simulink model "vienna_car_part2"  (R2019b)
settings: Solver=VariableStepAuto  StartTime=0.0  StopTime=100  RelTol=1e-3
values from neighbouring files (symbols this model uses):
  simulation_length_track = distance_A_B    [main.m]
  slope_of_track = 3    [main.m]
undefined symbols (not defined in the file or in its folder): air_density, drag_coefficient, equ_mass_of_rot_parts, gravity, mass, rolling_resistance_coefficient_0, rolling_resistance_coefficient_1, surface_area, wheel_radius
settings Model: Creator=jamil  LastModifiedBy=jamil
settings SolverCC: ZeroCrossAlgorithm=Adaptive
settings DebuggingCC: IgnoredZcDiagnostic=none

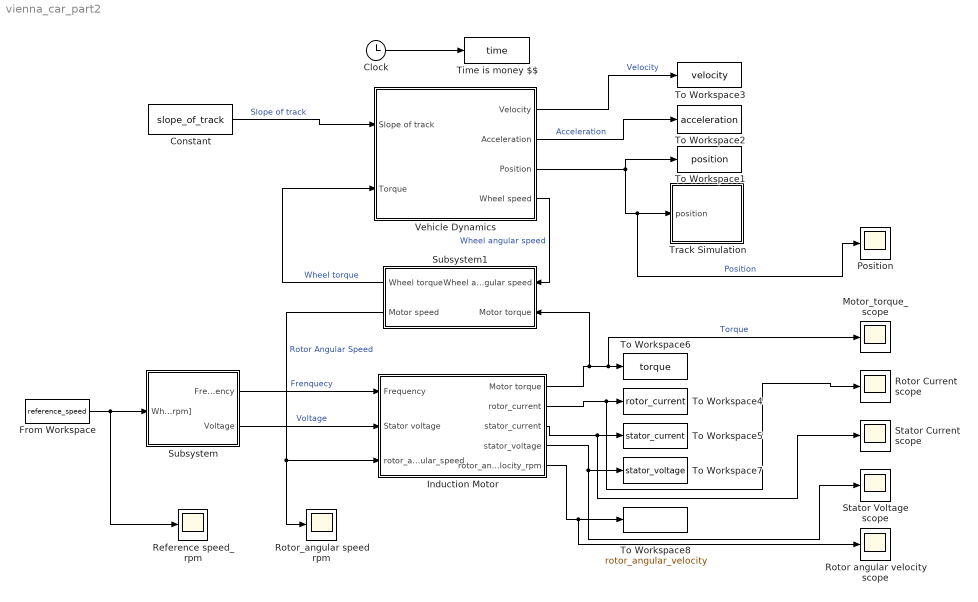
== system vienna_car_part2 ==
  Clock : Clock
  Constant : Constant  Value=slope_of_track
  From Workspace : FromWorkspace  VariableName=reference_speed  SampleTime=0
  Induction Motor : Subsystem
      mask Display: image('induction_motor_pic.jpg')
  Motor_torque_scope : Scope
  Position : Scope
  Reference speed_rpm : Scope
  "Rotor Current scope " : Scope
  Rotor angular velocity scope : Scope
  Rotor_angular speed rpm : Scope
  Stator Current scope : Scope
  Stator Voltage scope : Scope
  Subsystem : Subsystem
      mask Display: image('variable_speed_drive_pic.png')
  Subsystem1 : Subsystem
      mask Display: image('gearbox_pic.jpg'); % Use "Edit Image" on toolstrip to change.
  Time is money $$ : ToWorkspace  VariableName=time  SampleTime=-1
  To Workspace1 : ToWorkspace  VariableName=position  SampleTime=-1
  To Workspace2 : ToWorkspace  VariableName=acceleration  SampleTime=-1
  To Workspace3 : ToWorkspace  VariableName=velocity  SampleTime=-1
  To Workspace4 : ToWorkspace  VariableName=rotor_current  SampleTime=-1
  To Workspace5 : ToWorkspace  VariableName=stator_current  SampleTime=-1
  To Workspace6 : ToWorkspace  VariableName=torque  SampleTime=-1
  To Workspace7 : ToWorkspace  VariableName=stator_voltage  SampleTime=-1
  To Workspace8 : ToWorkspace  VariableName=rotor_angular_velocity  SampleTime=-1
  Track Simulation : Subsystem
  Vehicle Dynamics : Subsystem
      mask Display: image('car_dynamic_pic.jpg'); % Use "Edit Image" on toolstrip to change.
  wires:
  Vehicle Dynamics/2(Acceleration) -> To Workspace2/1  "Acceleration"
  Vehicle Dynamics/3(Position) -> Position/1, Track Simulation/1(position), To Workspace1/1  "Position"
  Constant/1 -> Vehicle Dynamics/1("Slope of track ")  "Slope of track"
  Vehicle Dynamics/1(Velocity) -> To Workspace3/1  "Velocity"
  Clock/1 -> Time is money $$/1
  Subsystem1/2(Motor speed) -> Rotor_angular speed rpm/1, Induction Motor/3("rotor_angular_speed ")  "Rotor Angular Speed"
  Induction Motor/1(Motor torque) -> Subsystem1/2(Motor torque), Motor_torque_scope/1, To Workspace6/1  "Torque"
  Subsystem/1(Frequency) -> Induction Motor/1("Frequency ")  "Frenquecy"
  Subsystem/2(Voltage) -> Induction Motor/2("Stator voltage ")  "Voltage"
  From Workspace/1 -> Reference speed_rpm/1, Subsystem/1(Wheel speed [rpm])
  Induction Motor/4(stator_voltage) -> Stator Voltage scope/1, To Workspace7/1
  Induction Motor/5(rotor_angular_velocity_rpm) -> Rotor angular velocity scope/1, To Workspace8/1
  Induction Motor/2(rotor_current) -> "Rotor Current scope "/1, To Workspace4/1
  Induction Motor/3(stator_current) -> Stator Current scope/1, To Workspace5/1
  Vehicle Dynamics/4(Wheel speed) -> Subsystem1/1(Wheel angular speed)  "Wheel angular speed"
  Subsystem1/1("Wheel torque ") -> Vehicle Dynamics/2(Torque)  "Wheel torque"

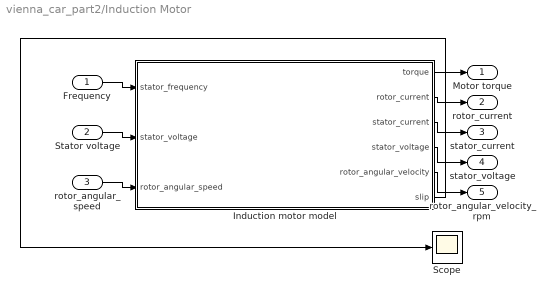
== system vienna_car_part2/Induction Motor ==
  "Frequency " : Inport
  "Stator voltage " : Inport  Port=2
  "rotor_angular_speed " : Inport  Port=3
  "Induction motor model " : MATLAB Function  TreatAsAtomicUnit=on
  Scope : Scope
  Motor torque : Outport
  rotor_current : Outport  Port=2
  stator_current : Outport  Port=3
  stator_voltage : Outport  Port=4
  rotor_angular_velocity_rpm : Outport  Port=5
  wires:
  "Induction motor model "/1(torque) -> Motor torque/1
  "Stator voltage "/1 -> "Induction motor model "/2("stator_voltage ")
  "rotor_angular_speed "/1 -> "Induction motor model "/3(rotor_angular_speed)
  "Induction motor model "/2(rotor_current) -> rotor_current/1
  "Induction motor model "/3(stator_current) -> stator_current/1
  "Induction motor model "/4(stator_voltage) -> stator_voltage/1
  "Frequency "/1 -> "Induction motor model "/1(stator_frequency)
  "Induction motor model "/5(rotor_angular_velocity) -> rotor_angular_velocity_rpm/1
  "Induction motor model "/6(slip) -> Scope/1

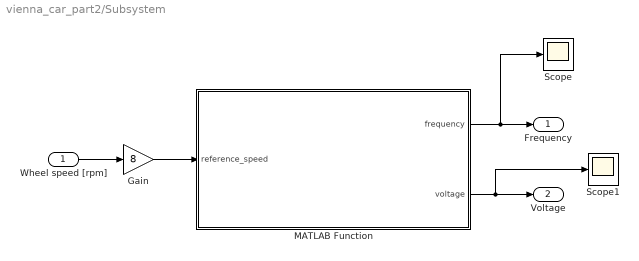
== system vienna_car_part2/Subsystem ==
  Wheel speed [rpm] : Inport
  Gain : Gain  Gain=8
  MATLAB Function : MATLAB Function  TreatAsAtomicUnit=on
  Scope : Scope
  Scope1 : Scope
  Frequency : Outport
  Voltage : Outport  Port=2
  wires:
  MATLAB Function/1(frequency) -> Scope/1, Frequency/1
  MATLAB Function/2(voltage) -> Scope1/1, Voltage/1
  Wheel speed [rpm]/1 -> Gain/1
  Gain/1 -> MATLAB Function/1(reference_speed)

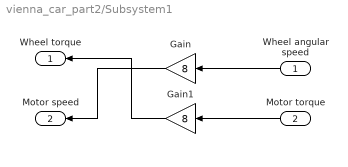
== system vienna_car_part2/Subsystem1 ==
  Wheel angular speed : Inport
  Motor torque : Inport  Port=2
  Gain : Gain  Gain=8
  Gain1 : Gain  Gain=8
  "Wheel torque " : Outport
  Motor speed : Outport  Port=2
  wires:
  Gain/1 -> Motor speed/1
  Wheel angular speed/1 -> Gain/1
  Gain1/1 -> "Wheel torque "/1
  Motor torque/1 -> Gain1/1

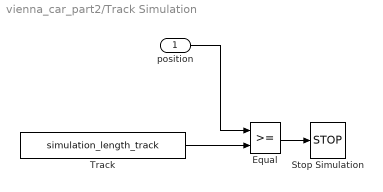
== system vienna_car_part2/Track Simulation ==
  position : Inport
  Equal : RelationalOperator  OutDataTypeStr=boolean  RndMeth=Simplest
  Stop Simulation : Stop
  "Track " : Constant  Value=simulation_length_track
  wires:
  Equal/1 -> Stop Simulation/1
  position/1 -> Equal/1
  "Track "/1 -> Equal/2

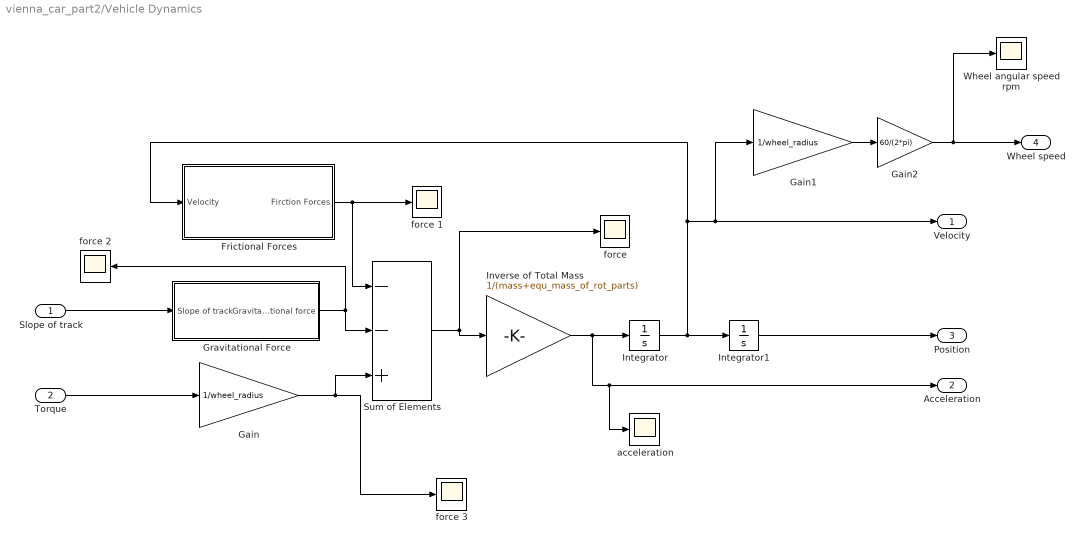
== system vienna_car_part2/Vehicle Dynamics ==
  "Slope of track " : Inport
  Torque : Inport  Port=2
  Frictional Forces : Subsystem
  Gain : Gain  Gain=1/wheel_radius
  Gain1 : Gain  Gain=1/wheel_radius
  Gain2 : Gain  Gain=60/(2*pi)
  Gravitational Force : Subsystem
  Integrator : Integrator
  Integrator1 : Integrator
  Inverse of Total Mass : Gain  Gain=1/(mass+equ_mass_of_rot_parts)
  Sum of Elements : Sum  Inputs=--+
  Wheel angular speed rpm : Scope
  acceleration : Scope
  force {,1..3} (4 alike) : Scope
  Velocity : Outport
  Acceleration : Outport  Port=2
  Position : Outport  Port=3
  Wheel speed : Outport  Port=4
  wires:
  Integrator1/1 -> Position/1
  Inverse of Total Mass/1 -> Integrator/1, acceleration/1, Acceleration/1
  Sum of Elements/1 -> Inverse of Total Mass/1, "force "/1
  Frictional Forces/1(Firction Forces) -> Sum of Elements/1, force 1/1
  "Slope of track "/1 -> Gravitational Force/1(Slope of track)
  Gravitational Force/1(Gravitational force) -> Sum of Elements/2, force 2/1
  Torque/1 -> Gain/1
  Gain/1 -> force 3/1, Sum of Elements/3
  Gain2/1 -> Wheel angular speed rpm/1, Wheel speed/1
  Integrator/1 -> Integrator1/1, Frictional Forces/1(Velocity), Gain1/1, Velocity/1
  Gain1/1 -> Gain2/1

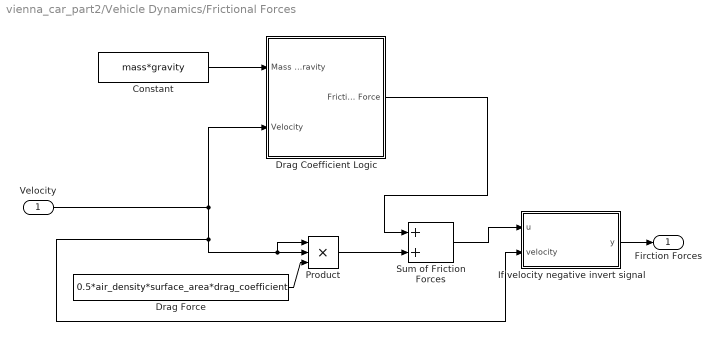
== system vienna_car_part2/Vehicle Dynamics/Frictional Forces ==
  Velocity : Inport
  Constant : Constant  Value=mass*gravity
  Drag Coefficient Logic : Subsystem
  Drag Force : Constant  Value=0.5*air_density*surface_area*drag_coefficient
  If velocity negative invert signal : MATLAB Function  TreatAsAtomicUnit=on
  Product : Product  Inputs=3
  Sum of Friction Forces : Sum
  Firction Forces : Outport
  wires:
  Drag Force/1 -> Product/3
  Constant/1 -> Drag Coefficient Logic/1("Mass and Gravity ")
  Drag Coefficient Logic/1(Friction Force) -> Sum of Friction Forces/1
  Velocity/1 -> Product/1, Product/2, If velocity negative invert signal/2(velocity), Drag Coefficient Logic/2(Velocity)
  Product/1 -> Sum of Friction Forces/2
  Sum of Friction Forces/1 -> If velocity negative invert signal/1(u)
  If velocity negative invert signal/1(y) -> Firction Forces/1

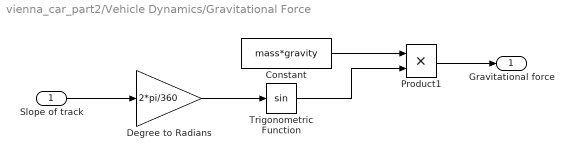
== system vienna_car_part2/Vehicle Dynamics/Gravitational Force ==
  Slope of track : Inport
  Constant : Constant  Value=mass*gravity
  Degree to Radians : Gain  Gain=2*pi/360
  Product1 : Product
  Trigonometric Function : Trigonometry
  Gravitational force : Outport
  wires:
  Product1/1 -> Gravitational force/1
  Constant/1 -> Product1/1
  Trigonometric Function/1 -> Product1/2
  Slope of track/1 -> Degree to Radians/1
  Degree to Radians/1 -> Trigonometric Function/1

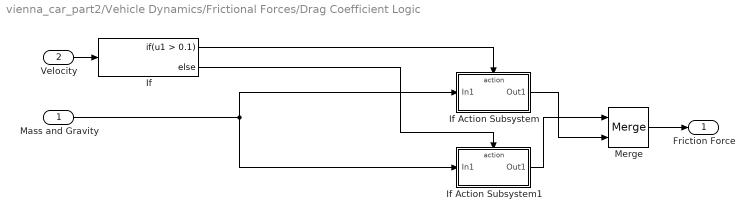
== system vienna_car_part2/Vehicle Dynamics/Frictional Forces/Drag Coefficient Logic ==
  "Mass and Gravity " : Inport
  Velocity : Inport  Port=2
  If : If  IfExpression=u1 > 0.1
  If Action Subsystem : Subsystem  TreatAsAtomicUnit=on
  If Action Subsystem1 : Subsystem  TreatAsAtomicUnit=on
  Merge : Merge
  Friction Force : Outport
  wires:
  If Action Subsystem/1(Out1) -> Merge/2
  If Action Subsystem1/1(Out1) -> Merge/1
  If/2 -> If Action Subsystem1/Action
  "Mass and Gravity "/1 -> If Action Subsystem/1(In1), If Action Subsystem1/1(In1)
  Merge/1 -> Friction Force/1
  If/1 -> If Action Subsystem/Action
  Velocity/1 -> If/1

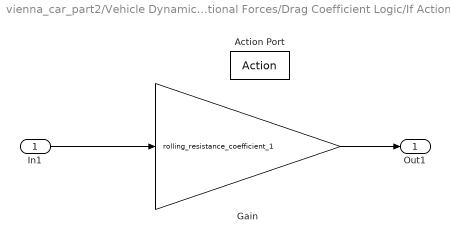
== system vienna_car_part2/Vehicle Dynamics/Frictional Forces/Drag Coefficient Logic/If Action Subsystem ==
  In1 : Inport
  Action Port : ActionPort  ActionPortLabel=if(u1 > 0.1)
  Gain : Gain  Gain=rolling_resistance_coefficient_1
  Out1 : Outport
  wires:
  In1/1 -> Gain/1
  Gain/1 -> Out1/1

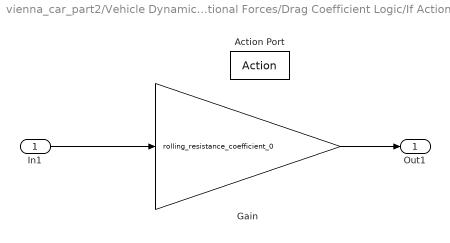
== system vienna_car_part2/Vehicle Dynamics/Frictional Forces/Drag Coefficient Logic/If Action Subsystem1 ==
  In1 : Inport
  Action Port : ActionPort  ActionPortLabel=else
  Gain : Gain  Gain=rolling_resistance_coefficient_0
  Out1 : Outport
  wires:
  In1/1 -> Gain/1
  Gain/1 -> Out1/1

== matlab function vienna_car_part2/Subsystem/MATLAB Function ==
  data: reference_speed input; frequency output; voltage output
function [frequency, voltage] = fcn(reference_speed)
frequency = reference_speed*2/60;
voltage = frequency;
end

== matlab function vienna_car_part2/Induction Motor/Induction motor model  ==
  data: stator_frequency input; torque output; stator_voltage input; rotor_angular_speed input; rotor_current output; stator_current output; stator_voltage output; rotor_angular_velocity output; slip output
function [torque, rotor_current, stator_current, stator_voltage, rotor_angular_velocity, slip] = fcn(stator_frequency, stator_voltage, rotor_angular_speed)
    % slip
    slip = (60*stator_frequency - rotor_angular_speed)/(60*stator_frequency);
    % Constant specs
    stator_resistance = 8.56*1e-3;
    stator_leakage_inductance = 0.06292 * 1e-3;
    mutual_inductance = 1.0122 * 1e-3;
    rotor_resistance = 10.20 *1e-3;
    rotor_leakage_inductance = 0.06709 * 1e-3;
    % Variable specs
    stator_voltage = stator_voltage/sqrt(3); % phase-phase -> % phase-neutral
    stator_reactance = stator_leakage_inductance * 2 * pi * stator_frequency * 1i;
    rotor_reactance = rotor_leakage_inductance * 2 * pi * stator_frequency * 1i;
    mutual_reactance = mutual_inductance * 2 * pi * stator_frequency * 1i;
    stator_impedance = stator_resistance + stator_reactance;
    rotor_impedance = rotor_resistance + rotor_reactance; 
    % Descriptive Equations
    equivalent_impedance = stator_impedance + (mutual_reactance*(((-slip +1)/slip)*rotor_resistance+rotor_impedance))/(mutual_reactance+(((-slip+1)/slip)*rotor_resistance+rotor_impedance));
    stator_current = stator_voltage/equivalent_impedance;
     % Calculus of torque
     rotor_current = stator_current - (stator_voltage-stator_current*stator_impedance)/(mutual_reactance);
     if (slip == 0 )
         torque = 0;
     else
         torque = (3*rotor_resistance*abs(rotor_current)^2)/(slip*stator_frequency*2*pi); %if s = 0 => binario  igual a 0
     end
     rotor_angular_velocity = (1-slip)*stator_frequency*60;
end

== matlab function vienna_car_part2/Vehicle Dynamics/Frictional Forces/If velocity negative invert signal ==
  data: u input; y output; velocity input
function y = fcn(u, velocity)
if (velocity < 0 )
    y = - u;
else
    y = u;
end
end
